simulink model "mechanical_model_sine_input"  (R2019b)
settings: Solver=FixedStepAuto  StartTime=0.0  StopTime=70  FixedStep=1e-3  RelTol=1e-3
undefined symbols (not defined in the file or in its folder): amplP, omegaP, symTf1, symTf2
settings Model: Creator=Guido  LastModifiedBy=pietr

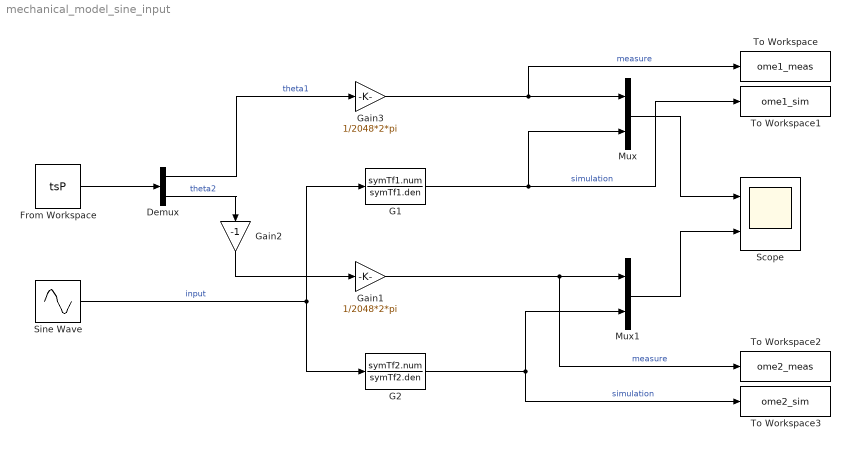
== system mechanical_model_sine_input ==
  Demux : Demux  Outputs=2
  From Workspace : FromWorkspace  VariableName=tsP  SampleTime=0
  G1 : TransferFcn  Numerator=symTf1.num  Denominator=symTf1.den
  G2 : TransferFcn  Numerator=symTf2.num  Denominator=symTf2.den
  Gain1 : Gain  Gain=1/2048*2*pi
  Gain2 : Gain  Gain=-1
  Gain3 : Gain  Gain=1/2048*2*pi
  Mux : Mux  Inputs=2
  Mux1 : Mux  Inputs=2
  Scope : Scope  NumInputPorts=2
  Sine Wave : Sin  Amplitude=amplP  Frequency=omegaP  SampleTime=0
  To Workspace : ToWorkspace  VariableName=ome1_meas  SaveFormat=Timeseries  SampleTime=-1
  To Workspace1 : ToWorkspace  VariableName=ome1_sim  SaveFormat=Timeseries  SampleTime=-1
  To Workspace2 : ToWorkspace  VariableName=ome2_meas  SaveFormat=Timeseries  SampleTime=-1
  To Workspace3 : ToWorkspace  VariableName=ome2_sim  SaveFormat=Timeseries  SampleTime=-1
  wires:
  Gain1/1 -> To Workspace2/1, Mux1/1  "measure"
  Demux/1 -> Gain3/1  "theta1"
  Demux/2 -> Gain2/1  "theta2"
  Mux/1 -> Scope/1
  Mux1/1 -> Scope/2
  From Workspace/1 -> Demux/1
  Gain2/1 -> Gain1/1
  Gain3/1 -> To Workspace/1, Mux/1  "measure"
  G1/1 -> Mux/2, To Workspace1/1  "simulation"
  Sine Wave/1 -> G2/1, G1/1  "input"
  G2/1 -> To Workspace3/1, Mux1/2  "simulation"
